simulink model "fuzzymodel"  (R2019b)
settings: Solver=ode45  StartTime=0.0  StopTime=0.3  RelTol=1e-3
libraries: powerlib x9, fuzblock x1, re_lib x1, powerlib_meascontrol x1
settings Model: Creator=risha  LastModifiedBy=risha

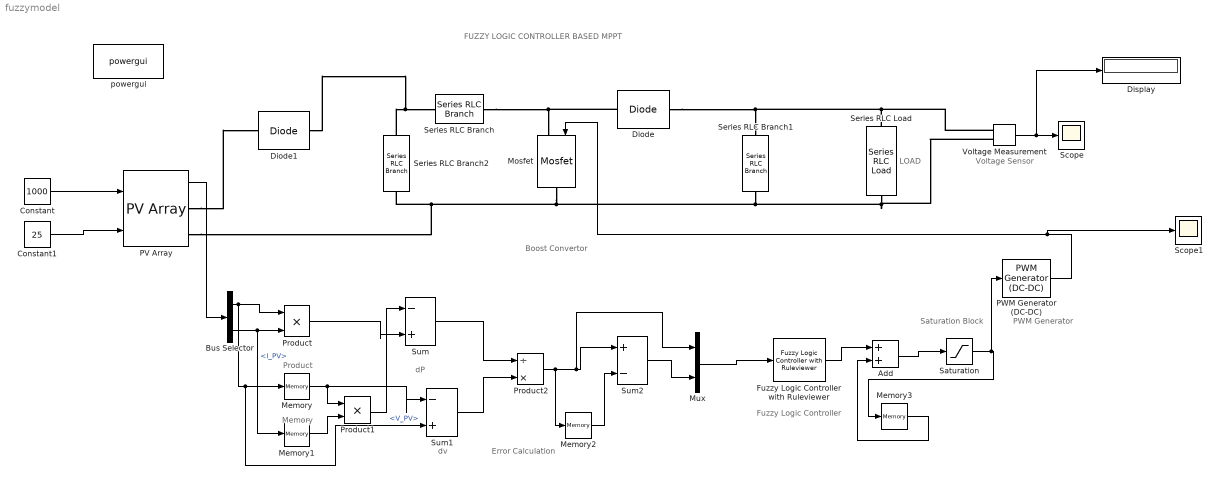
== system fuzzymodel ==
  note: Voltage Sensor
  note: FUZZY LOGIC CONTROLLER BASED MPPT
  note: LOAD
  note: PWM Generator
  note: Saturation Block
  note: Boost Convertor
  note: Fuzzy Logic Controller
  note: Error Calculation
  note: Memory
  note: Product
  note: dv
  note: dP
  Add : Sum
  Bus Selector : BusSelector  OutputSignals=V_PV,I_PV
  Constant : Constant  Value=1000
  Constant1 : Constant  Value=25
  Diode : powerlib/Power Electronics/Diode  Ron=0.001  Lon=0  Vf=0.8  IC=0  UseSnubber=0  Rs=500  Cs=250e-9  Measurements=off
      settings: SourceProductName=Simscape Electrical
  Diode1 : powerlib/Power Electronics/Diode  Ron=0.001  Lon=0  Vf=0.8  IC=0  UseSnubber=0  Rs=500  Cs=250e-9  Measurements=off
      settings: SourceProductName=Simscape Electrical
  Display : Display
  Fuzzy Logic Controller with Ruleviewer : fuzblock/Fuzzy Logic  Controller  with Ruleviewer  fismatrix=mppt  Ts=0.01
  Memory{,1..3} (4 alike) : Memory
  Mosfet : powerlib/Power Electronics/Mosfet  Ron=0.1  Lon=0  Rd=0.01  Vfd=0  IC=0  Rs=1e5  Cs=inf  Measurements=off
      settings: SourceProductName=Simscape Electrical
  Mux : Mux  Inputs=2
  PV Array : re_lib/Solar/PV Array  Npar=1  Nser=1  PlotType=one module @ 25 deg.C & specified irradiances  S_vec=[800]  Temp_C_vec="[ 45 25  ]"  ModuleName=Kyocera Solar KC130TM  PlotWhenSelected=off  Pm=130.064  Ncell=36  Voc=21.9  Isc=8.02  Vm=17.6  Im=7.39  beta_Voc_pc=-0.35502  alpha_Isc_pc=0.06  beta_Voc=-0.07775  alpha_Isc=0.004812  IL=8.0428  I0=2.2655e-10  nI=0.97611  Rsh=78.0854  Rs=0.22151  BAL=on  Tc=1e-6  Tfilter=5e-5
      settings: SourceProductName=Simscape Electrical
  PWM Generator (DC-DC) : powerlib_meascontrol/Pulse & Signal Generators/PWM Generator (DC-DC)  Fsw=5000  Ts=0
      settings: SourceProductName=Simscape Electrical
  Product : Product
  Product1 : Product
  Product2 : Product  Inputs=/*
  Saturation : Saturate
  Scope : Scope
  Scope1 : Scope
  Series RLC Branch : powerlib/Elements/Series RLC Branch  LConnTagsString=__new0  RConnTagsString=__new0  BranchType=L  Resistance=1  Inductance=1e-4  SetiL0=off  InitialCurrent=0  Capacitance=1e-6  Setx0=off  InitialVoltage=0  Measurements=None
      settings: SourceProductName=Simscape Electrical
  Series RLC Branch1 : powerlib/Elements/Series RLC Branch  LConnTagsString=__new0  RConnTagsString=__new0  BranchType=C  Resistance=1  Inductance=1e-4  SetiL0=off  InitialCurrent=0  Capacitance=50e-6  Setx0=off  InitialVoltage=0  Measurements=None
      settings: SourceProductName=Simscape Electrical
  Series RLC Branch2 : powerlib/Elements/Series RLC Branch  LConnTagsString=__new0  RConnTagsString=__new0  BranchType=C  Resistance=1  Inductance=1e-4  SetiL0=off  InitialCurrent=0  Capacitance=4000e-6  Setx0=off  InitialVoltage=0  Measurements=None
      settings: SourceProductName=Simscape Electrical
  Series RLC Load : powerlib/Elements/Series RLC Load  LConnTagsString=a  RConnTagsString=__new0  NominalVoltage=30  NominalFrequency=50  ActivePower=120  InductivePower=0  CapacitivePower=0  Setx0=off  InitialVoltage=0  SetiL0=off  InitialCurrent=0  Measurements=None  LoadType=constant Z
      settings: SourceProductName=Simscape Electrical
  Sum : Sum  Inputs=|-+
  Sum1 : Sum  Inputs=|-+
  Sum2 : Sum  Inputs=|+-
  Voltage Measurement : powerlib/Measurements/Voltage Measurement  PhasorSimulation=off  OutputType=Complex  PSBequivalent=0
      settings: SourceProductName=Simscape Electrical
  powergui : powerlib/powergui  Priority=1  SimulationMode=Discrete  SampleTime=50e-6  frequency=60  Iterations=50  frequencyindice=0  Pbase=100e6  ErrMax=1e-4  UnitsV=kV  UnitsW=MW  buscounter=0  FunctionMessages=off  echomessages=off  EnableUseOfTLC=off  CurrentSourceSwitches=off  DisableSnubberDevices=off  DisableRonSwitches=off  DisableVfSwitches=off  DisplayEquations=off  AutomaticDiscreteSolvers=off  SolverType=Tustin/Backward Euler (TBE)  Interpol=off  ExternalGateDelay=off  methode=off  Ts=100  x0status=blocks  SPID=on  SwTol=0  HookPort=off  NonlinearTolerance=1e-4  nMaxIteration=100  ContinueOnMaxIteration=off  RestoreLinks=warning  ResistiveCurrentMeasurement=off  Frange=[0:2:500]  Ylog=off  Xlog=on  ShowGrid=off  save=off  variable=ZData  structure=0  ZoomFFT=off  StartTime=0.0  cycles=1  DisplayStyle=1  fundamental=60  FreqAxis=off  MaxFrequency=1000  frequencyindicesteady=1  RmsSteady=1  display=off
      settings: SourceProductName=Simscape Electrical
  wires:
  Constant/1 -> PV Array/1
  Constant1/1 -> PV Array/2
  PV Array/1 -> Bus Selector/1
  Product/1 -> Sum/2
  Memory/1 -> Sum1/1, Product1/1
  Memory1/1 -> Product1/2
  Product1/1 -> Sum/1
  Bus Selector/1 -> Sum1/2, Memory/1, Product/1  "<V_PV>"
  Bus Selector/2 -> Memory1/1, Product/2  "<I_PV>"
  Sum/1 -> Product2/1
  Sum1/1 -> Product2/2
  Product2/1 -> Memory2/1, Mux/1, Sum2/1
  Memory2/1 -> Sum2/2
  Sum2/1 -> Mux/2
  Mux/1 -> Fuzzy Logic Controller with Ruleviewer/1
  Add/1 -> Saturation/1
  Saturation/1 -> PWM Generator (DC-DC)/1, Memory3/1
  Memory3/1 -> Add/2
  PWM Generator (DC-DC)/1 -> Scope1/1, Mosfet/1
  Voltage Measurement/1 -> Display/1, Scope/1
  Fuzzy Logic Controller with Ruleviewer/1 -> Add/1
  connections:
  Series RLC Branch/RConn1 -- Diode/LConn1 -- Mosfet/LConn1
  Series RLC Load/LConn1 -- Voltage Measurement/LConn1 -- Diode/RConn1 -- Series RLC Branch1/LConn1
  Series RLC Branch2/LConn1 -- Diode1/RConn1 -- Series RLC Branch/LConn1
  Mosfet/RConn1 -- Voltage Measurement/LConn2 -- Series RLC Load/RConn1 -- Series RLC Branch1/RConn1 -- PV Array/RConn2 -- Series RLC Branch2/RConn1
  PV Array/RConn1 -- Diode1/LConn1
